simulink model "QuadControlSim"  (R2024b)
settings: Solver=FixedStepAuto  StartTime=0.0  StopTime=15  FixedStep=0.005  RelTol=1e-3
InitFcn:
  | R = 10; % Test Variable
values from neighbouring files (symbols this model uses):
  k = reshape(k,3,6)    [Initialization.m]
  p_Ref = trajMinSnap.p    [Initialization.m]
  psi_Ref = trajMinSnap.psi .* 180/pi    [Initialization.m]
  quad_X500 = quad_X500    [Initialization.m]
  t_Vec = trajMinSnap.t    [Initialization.m]
undefined symbols (not defined in the file or in its folder): kTemp
libraries: slpidlib x6, aerolibconvert2 x3, shared6dof x1, aerolibanimutils x1
settings Model: Creator=tdawg  LastModifiedBy=tdawg
settings SolverCC: ZeroCrossAlgorithm=Adaptive
settings DataIOCC: ReturnWorkspaceOutputs=off
settings DebuggingCC: IgnoredZcDiagnostic=none

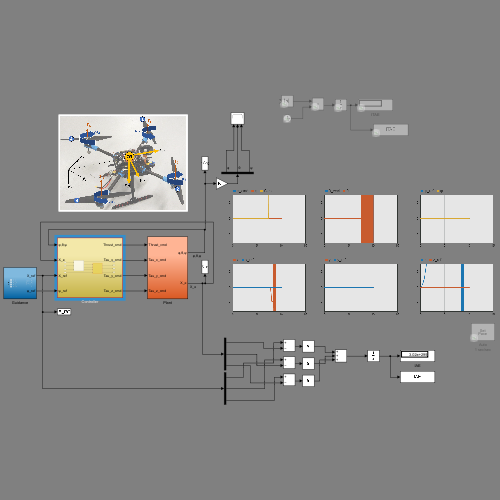
[thumbnail: Simulink's stored preview of the top-level diagram]
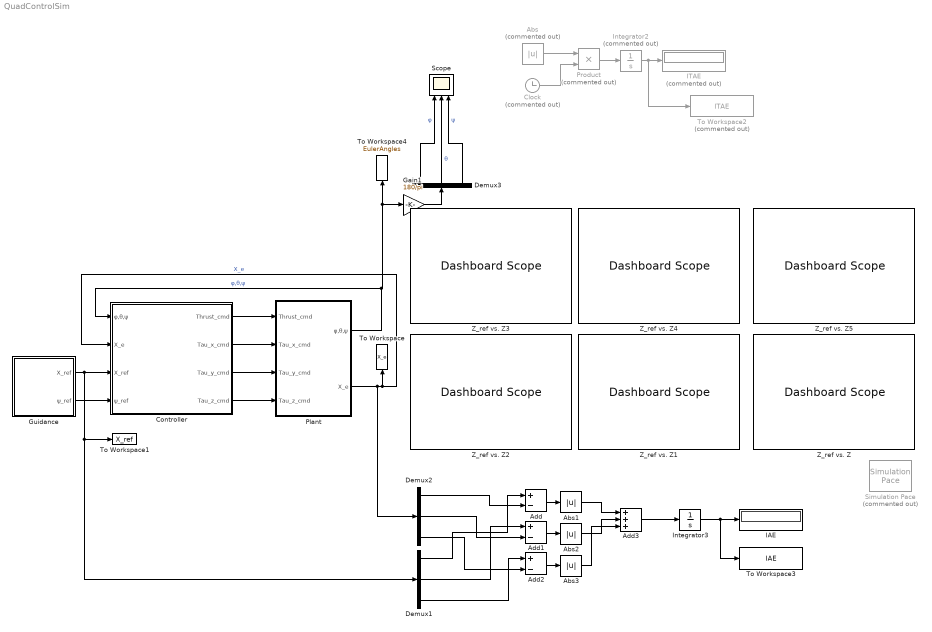
== system QuadControlSim ==
  Abs : Abs  Commented=on  SaturateOnIntegerOverflow=off
  Abs1 : Abs  SaturateOnIntegerOverflow=off
  Abs2 : Abs  SaturateOnIntegerOverflow=off
  Abs3 : Abs  SaturateOnIntegerOverflow=off
  Add : Sum  Inputs=+-
  Add1 : Sum  Inputs=+-
  Add2 : Sum  Inputs=+-
  Add3 : Sum  Inputs=+++
  Clock : Clock  Commented=on
  Controller : Subsystem
  Demux1 : Demux  Outputs=3
  Demux2 : Demux  Outputs=3
  Demux3 : Demux  Outputs=3
  Gain1 : Gain  Gain=180/pi
  Guidance : Subsystem
  IAE : Display
  ITAE : Display  Commented=on
  Integrator2 : Integrator  Commented=on
  Integrator3 : Integrator
  Plant : Subsystem
  Product : Product  Commented=on
  Scope : Scope  NumInputPorts=3
  Simulation Pace : aerolibanimutils/Simulation Pace  Commented=on  SimulationPace=1  SleepMode=Auto  OutputPaceError=off  SampleTime=1/200
  To Workspace : ToWorkspace  VariableName=X_e  SampleTime=-1
  To Workspace1 : ToWorkspace  VariableName=X_ref  SampleTime=-1
  To Workspace2 : ToWorkspace  Commented=on  VariableName=ITAE  SampleTime=-1
  To Workspace3 : ToWorkspace  VariableName=IAE  SampleTime=-1
  To Workspace4 : ToWorkspace  VariableName=EulerAngles  SampleTime=-1
  Z_ref vs. Z{,1..5} (6 alike) : DashboardScope
  wires:
  Guidance/2(ψ_ref) -> Controller/4(ψ_ref)
  Controller/1(Thrust_cmd) -> Plant/1(Thrust_cmd)
  Controller/2(Tau_x_cmd) -> Plant/2(Tau_x_cmd)
  Controller/3(Tau_y_cmd) -> Plant/3(Tau_y_cmd)
  Controller/4(Tau_z_cmd) -> Plant/4(Tau_z_cmd)
  Plant/1(φ,θ,ψ) -> Controller/1(φ,θ,ψ), To Workspace4/1, Gain1/1  "φ,θ,ψ"
  Plant/2(X_e) -> Demux2/1, Controller/2(X_e), To Workspace/1  "X_e"
  Integrator2/1 -> To Workspace2/1, ITAE/1
  Product/1 -> Integrator2/1
  Abs/1 -> Product/1
  Clock/1 -> Product/2
  Demux3/3 -> Scope/3  "ψ"
  Demux3/2 -> Scope/2  "θ"
  Demux3/1 -> Scope/1  "φ"
  Gain1/1 -> Demux3/1
  Add3/1 -> Integrator3/1
  Integrator3/1 -> To Workspace3/1, IAE/1
  Demux1/3 -> Add2/1
  Demux1/2 -> Add1/1
  Demux1/1 -> Add/1
  Demux2/3 -> Add2/2
  Demux2/2 -> Add1/2
  Demux2/1 -> Add/2
  Guidance/1(X_ref) -> Demux1/1, To Workspace1/1, Controller/3(X_ref)
  Add/1 -> Abs1/1
  Add1/1 -> Abs2/1
  Add2/1 -> Abs3/1
  Abs1/1 -> Add3/1
  Abs2/1 -> Add3/2
  Abs3/1 -> Add3/3

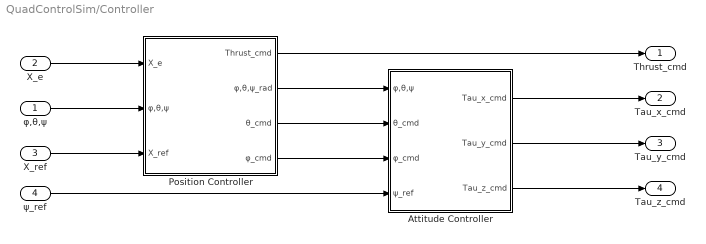
== system QuadControlSim/Controller ==
  φ,θ,ψ : Inport
  X_e : Inport  Port=2
  X_ref : Inport  Port=3
  ψ_ref : Inport  Port=4
  Attitude Controller : Subsystem
  Position Controller : Subsystem
  Thrust_cmd : Outport
  Tau_x_cmd : Outport  Port=2
  Tau_y_cmd : Outport  Port=3
  Tau_z_cmd : Outport  Port=4
  wires:
  Position Controller/4(φ_cmd) -> Attitude Controller/3(φ_cmd)
  Position Controller/2(φ,θ,ψ_rad) -> Attitude Controller/1(φ,θ,ψ)
  Position Controller/3(θ_cmd) -> Attitude Controller/2(θ_cmd)
  Position Controller/1(Thrust_cmd) -> Thrust_cmd/1
  Attitude Controller/1(Tau_x_cmd) -> Tau_x_cmd/1
  Attitude Controller/2(Tau_y_cmd) -> Tau_y_cmd/1
  Attitude Controller/3(Tau_z_cmd) -> Tau_z_cmd/1
  X_e/1 -> Position Controller/1(X_e)
  φ,θ,ψ/1 -> Position Controller/2(φ,θ,ψ)
  X_ref/1 -> Position Controller/3(X_ref)
  ψ_ref/1 -> Attitude Controller/4(ψ_ref)

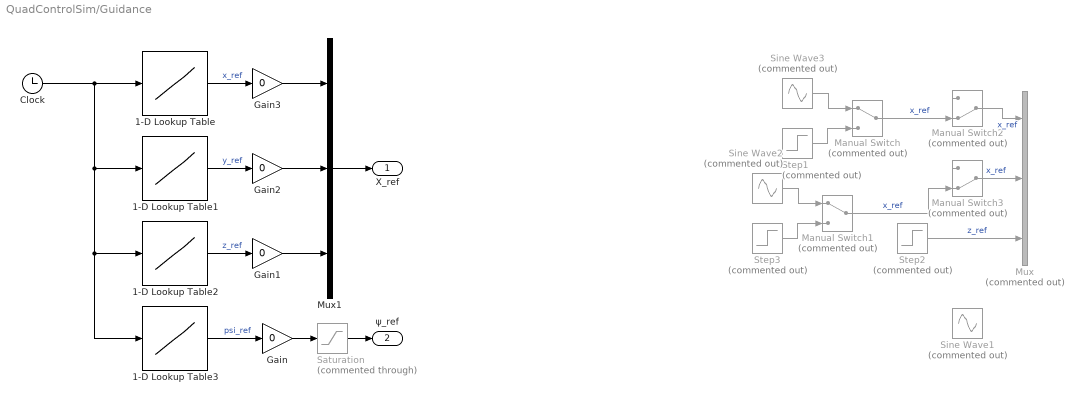
== system QuadControlSim/Guidance ==
  1-D Lookup Table : Lookup_n-D  NumberOfTableDimensions=1  BreakpointsForDimension1=t_Vec  Table=p_Ref(1,:)  InternalRulePriority=Speed  RndMeth=Simplest
  1-D Lookup Table1 : Lookup_n-D  NumberOfTableDimensions=1  BreakpointsForDimension1=t_Vec  Table=p_Ref(2,:)  InternalRulePriority=Speed  RndMeth=Simplest
  1-D Lookup Table2 : Lookup_n-D  NumberOfTableDimensions=1  BreakpointsForDimension1=t_Vec  Table=p_Ref(3,:)  InternalRulePriority=Speed  RndMeth=Simplest
  1-D Lookup Table3 : Lookup_n-D  NumberOfTableDimensions=1  BreakpointsForDimension1=t_Vec  Table=psi_Ref  InternalRulePriority=Speed  RndMeth=Simplest
  Clock : Clock
  Gain{,1..3} (4 alike) : Gain  Gain=0
  Manual Switch : ManualSwitch  Commented=on
  Manual Switch1 : ManualSwitch  Commented=on
  Manual Switch2 : ManualSwitch  Commented=on  CurrentSetting=0
  Manual Switch3 : ManualSwitch  Commented=on  CurrentSetting=0
  Mux : Mux  Commented=on  Inputs=3
  Mux1 : Mux  Inputs=3
  Saturation : Saturate  Commented=through  UpperLimit=175  LowerLimit=-175
  Sine Wave1 : Sin  Commented=on  Amplitude=0  SampleTime=0
  Sine Wave2 : Sin  Commented=on  Frequency=0.5  Phase=pi/2  SampleTime=0
  Sine Wave3 : Sin  Commented=on  Frequency=0.5  SampleTime=0
  Step1 : Step  Commented=on  Time=5  SampleTime=0
  Step2 : Step  Commented=on  After=-2  SampleTime=0
  Step3 : Step  Commented=on  Time=10  SampleTime=0
  X_ref : Outport
  ψ_ref : Outport  Port=2
  wires:
  Step2/1 -> Mux/3  "z_ref"
  Sine Wave3/1 -> Manual Switch/1
  Step1/1 -> Manual Switch/2
  Manual Switch/1 -> Manual Switch2/2  "x_ref"
  Step3/1 -> Manual Switch1/2
  Sine Wave2/1 -> Manual Switch1/1
  Manual Switch1/1 -> Manual Switch3/2  "x_ref"
  Manual Switch2/1 -> Mux/1  "x_ref"
  Manual Switch3/1 -> Mux/2  "x_ref"
  Clock/1 -> 1-D Lookup Table3/1, 1-D Lookup Table2/1, 1-D Lookup Table1/1, 1-D Lookup Table/1
  1-D Lookup Table/1 -> Gain3/1  "x_ref"
  1-D Lookup Table1/1 -> Gain2/1  "y_ref"
  1-D Lookup Table2/1 -> Gain1/1  "z_ref"
  1-D Lookup Table3/1 -> Gain/1  "psi_ref"
  Mux1/1 -> X_ref/1
  Saturation/1 -> ψ_ref/1
  Gain/1 -> Saturation/1
  Gain2/1 -> Mux1/2
  Gain3/1 -> Mux1/1
  Gain1/1 -> Mux1/3

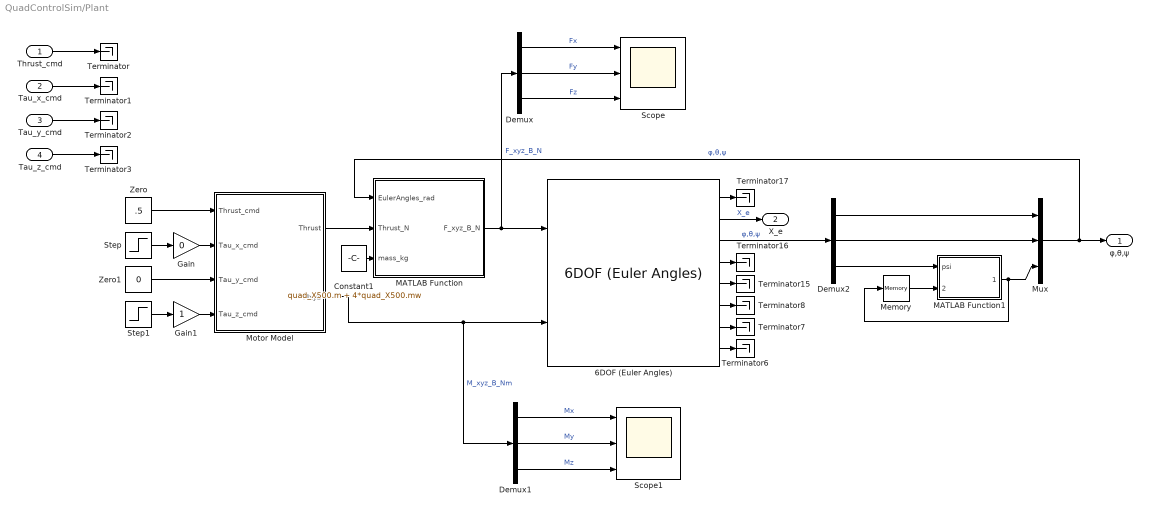
== system QuadControlSim/Plant ==
  Thrust_cmd : Inport
  Tau_x_cmd : Inport  Port=2
  Tau_y_cmd : Inport  Port=3
  Tau_z_cmd : Inport  Port=4
  6DOF (Euler Angles) : shared6dof/6DOF (Euler Angles)  units=Metric (MKS)  mtype=Fixed  rep=Euler Angles  xme_0=[0 0 0]  Vm_0=[0 0 0]  eul_0=[0 0 0]  pm_0=[0 0 0]  mass_0=quad_X500.m + 4*quad_X500.mw  mass_e=0.5  mass_f=2.0  inertia=quad_X500.I  inertia_e=eye(3)  inertia_f=2*eye(3)  k_quat=1  vre_flag=on  abi_flag=off  aMode=0  xme_statename=''  Vm_statename=''  eul_statename=''  quat_statename=''  pm_statename=''  mass_statename=''
  Constant1 : Constant  Value=quad_X500.m + 4*quad_X500.mw
  Demux : Demux  Outputs=3
  Demux1 : Demux  Outputs=3
  Demux2 : Demux  Outputs=3
  Gain : Gain  Gain=0
  Gain1 : Gain
  MATLAB Function : MATLAB Function  TreatAsAtomicUnit=on
  MATLAB Function1 : MATLAB Function  TreatAsAtomicUnit=on
  Memory : Memory
  Motor Model : Subsystem
  Mux : Mux  Inputs=3'
  Scope : Scope  NumInputPorts=3
  Scope1 : Scope  NumInputPorts=3
  Step : Step  Time=7.5  After=0.05  SampleTime=0
  Step1 : Step  Time=7.5  After=0.05  SampleTime=0
  Terminator{,1..3,6..8,15..17} (10 alike) : Terminator
  Zero : Constant  Value=.5  OutDataTypeStr=Inherit: Inherit via back propagation
  Zero1 : Constant  Value=0  OutDataTypeStr=Inherit: Inherit via back propagation
  φ,θ,ψ : Outport
  X_e : Outport  Port=2
  wires:
  6DOF (Euler Angles)/4 -> Terminator16/1
  Constant1/1 -> MATLAB Function/3(mass_kg)
  6DOF (Euler Angles)/6 -> Terminator8/1
  6DOF (Euler Angles)/8 -> Terminator6/1
  MATLAB Function/1(F_xyz_B_N) -> Demux/1, 6DOF (Euler Angles)/1  "F_xyz_B_N"
  6DOF (Euler Angles)/7 -> Terminator7/1
  6DOF (Euler Angles)/5 -> Terminator15/1
  6DOF (Euler Angles)/1 -> Terminator17/1
  6DOF (Euler Angles)/2 -> X_e/1  "X_e"
  Motor Model/1(Thrust) -> MATLAB Function/2(Thrust_N)
  Motor Model/2(Mxyz) -> Demux1/1, 6DOF (Euler Angles)/2  "M_xyz_B_Nm"
  Demux/1 -> Scope/1  "Fx"
  Demux/2 -> Scope/2  "Fy"
  Demux/3 -> Scope/3  "Fz"
  Demux1/1 -> Scope1/1  "Mx"
  Demux1/2 -> Scope1/2  "My"
  Demux1/3 -> Scope1/3  "Mz"
  Demux2/3 -> MATLAB Function1/1(psi)
  MATLAB Function1/1(psi_corrected) -> Mux/3, Memory/1
  Memory/1 -> MATLAB Function1/2(psi_prev)
  6DOF (Euler Angles)/3 -> Demux2/1  "φ,θ,ψ"
  Demux2/2 -> Mux/2
  Demux2/1 -> Mux/1
  Mux/1 -> MATLAB Function/1(EulerAngles_rad), φ,θ,ψ/1  "φ,θ,ψ"
  Thrust_cmd/1 -> Terminator/1
  Tau_x_cmd/1 -> Terminator1/1
  Tau_y_cmd/1 -> Terminator2/1
  Tau_z_cmd/1 -> Terminator3/1
  Zero/1 -> Motor Model/1(Thrust_cmd)
  Zero1/1 -> Motor Model/3(Tau_y_cmd)
  Step/1 -> Gain/1
  Gain/1 -> Motor Model/2(Tau_x_cmd)
  Step1/1 -> Gain1/1
  Gain1/1 -> Motor Model/4(Tau_z_cmd)

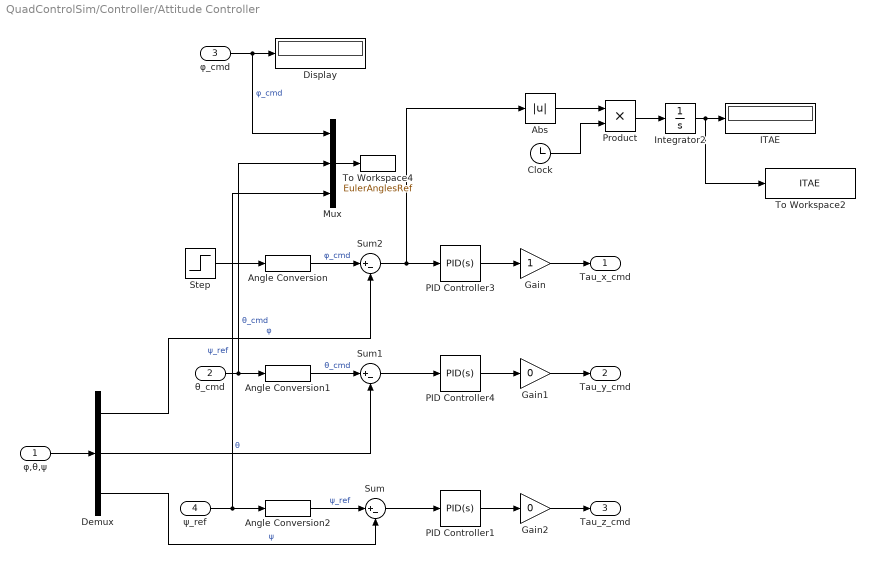
== system QuadControlSim/Controller/Attitude Controller ==
  φ,θ,ψ : Inport
  θ_cmd : Inport  Port=2
  φ_cmd : Inport  Port=3
  ψ_ref : Inport  Port=4
  Abs : Abs  SaturateOnIntegerOverflow=off
  Angle Conversion : aerolibconvert2/Angle Conversion  IU=deg  OU=rad
  Angle Conversion1 : aerolibconvert2/Angle Conversion  IU=deg  OU=rad
  Angle Conversion2 : aerolibconvert2/Angle Conversion  IU=deg  OU=rad
  Clock : Clock
  Demux : Demux  Outputs=3
  Display : Display
  Gain : Gain
  Gain1 : Gain  Gain=0
  Gain2 : Gain  Gain=0
  ITAE : Display
  Integrator2 : Integrator
  Mux : Mux  Inputs=3
  PID Controller1 : slpidlib/PID Controller  Controller=PID  Form=Parallel  TimeDomain=Continuous-time  UseExternalTs=off  SampleTime=-1  IntegratorMethod=Forward Euler  FilterMethod=Forward Euler  ControllerParametersSource=internal  P=k(1,3)  I=k(2,3)  UseKiTs=off  D=k(3,3)  UseExternalDerivativeSource=off  N=100  UseFilter=on  TunerSelectOption=Transfer Function Based (PID Tuner App)  InitialConditionSource=internal  InitialConditionForIntegrator=0  InitialConditionForFilter=0  DifferentiatorICPrevScaledInput=0  ExternalReset=none  TrackingMode=off  Kt=1  LimitOutput=on  SatLimitsSource=internal  UpperSaturationLimit=0.07  LowerSaturationLimit=-0.07  LinearizeAsGain=off  AntiWindupMode=clamping  Kb=0.25  LimitIntegrator=off  UpperIntegratorSaturationLimit=inf  LowerIntegratorSaturationLimit=-inf  POutMin=[]  POutMax=[]  IOutMin=[]  IOutMax=[]  DOutMin=[]  DOutMax=[]  NOutMin=[]  NOutMax=[]  SumOutMin=[]  SumOutMax=[]  SaturationOutMin=[]  SaturationOutMax=[]  PParamMin=[]  PParamMax=[]  IParamMin=[]  IParamMax=[]  DParamMin=[]  DParamMax=[]  NParamMin=[]  NParamMax=[]  KbParamMin=[]  KbParamMax=[]  KtParamMin=[]  KtParamMax=[]  KbOutMin=[]  KbOutMax=[]  KtOutMin=[]  KtOutMax=[]  IntegratorOutMin=[]  IntegratorOutMax=[]  FilterOutMin=[]  FilterOutMax=[]  SumI1OutMin=[]  SumI1OutMax=[]  SumI2OutMin=[]  SumI2OutMax=[]  SumI3OutMin=[]  SumI3OutMax=[]  SumI4OutMin=[]  SumI4OutMax=[]  SumDOutMin=[]  SumDOutMax=[]  DifferentiatorOutMin=[]  DifferentiatorOutMax=[]  FilterDiffOutCoefMin=[]  FilterDiffOutCoefMax=[]  ReciprocalOutMin=[]  ReciprocalOutMax=[]  SumDenOutMin=[]  SumDenOutMax=[]  SumNumOutMin=[]  SumNumOutMax=[]  DivideOutMin=[]  DivideOutMax=[]  UdiffTsProdOutMin=[]  UdiffTsProdOutMax=[]  NTsProdOutMin=[]  NTsProdOutMax=[]  UintegralTsProdOutMin=[]  UintegralTsProdOutMax=[]  UngainTsProdOutMin=[]  UngainTsProdOutMax=[]  ClampingZeroOutDataTypeStr=Inherit: Inherit via back propagation  ClampingZeroOutMin=[]  ClampingZeroOutMax=[]  FilterDenConstantOutDataTypeStr=Inherit: Inherit via back propagation  FilterDenConstantOutMin=[]  FilterDenConstantOutMax=[]  PCopyOutDataTypeStr=Inherit: Inherit via back propagation  PCopyOutMin=[]  PCopyOutMax=[]  NCopyOutDataTypeStr=Inherit: Inherit via back propagation  NCopyOutMin=[]  NCopyOutMax=[]  IntegratorContinuousStateAttributes=''  IntegratorStateMustResolveToSignalObject=off  IntegratorRTWStateStorageClass=Auto  FilterContinuousStateAttributes=''  FilterStateMustResolveToSignalObject=off  FilterRTWStateStorageClass=Auto  ParallelPVariant=InternalParameters  IdealPVariant=Disabled  IVariant=InternalParameters  DVariant=InternalParameters  IntegratorVariant=Continuous  SatVariant=Enabled  AWVariant=ContClampingParallel  PCopyVariant=Disabled  TRVariant=Disabled  FdbkBlocksVariant=Forward  IdealPFdbkVariant=Disabled  SatFdbkVariant=Disabled  DerivativeFilterVariant=ContFilter  NVariant=InternalParameters  NCopyVariant=Disabled  FilterICVariant=InternalICsFilter  IntegratorICVariant=InternalICs  ExternalResetVariant=Disabled  TRSumVariant=Passthrough  SumFdbkVariant=Disabled  SumVariant=Sum_PID  TsampFilterVariant=InternalTs  TsampNgainVariant=Passthrough  TsampIntegralVariant=Disabled_SignalSpec  ExternalSaturationOutDataTypeStr=Inherit: Same as second input  DerivativeSourceVariant=ErrorSignal  PreIntVariant=InternalPreInt
  PID Controller3 : slpidlib/PID Controller  Controller=PID  Form=Parallel  TimeDomain=Continuous-time  UseExternalTs=off  SampleTime=-1  IntegratorMethod=Forward Euler  FilterMethod=Forward Euler  ControllerParametersSource=internal  P=kTemp(1)  I=kTemp(2)  UseKiTs=off  D=kTemp(3)  UseExternalDerivativeSource=off  N=100  UseFilter=on  TunerSelectOption=Transfer Function Based (PID Tuner App)  InitialConditionSource=internal  InitialConditionForIntegrator=0  InitialConditionForFilter=0  DifferentiatorICPrevScaledInput=0  ExternalReset=none  TrackingMode=off  Kt=1  LimitOutput=on  SatLimitsSource=internal  UpperSaturationLimit=0.05  LowerSaturationLimit=-0.05  LinearizeAsGain=off  AntiWindupMode=clamping  Kb=0.25  LimitIntegrator=off  UpperIntegratorSaturationLimit=inf  LowerIntegratorSaturationLimit=-inf  POutMin=[]  POutMax=[]  IOutMin=[]  IOutMax=[]  DOutMin=[]  DOutMax=[]  NOutMin=[]  NOutMax=[]  SumOutMin=[]  SumOutMax=[]  SaturationOutMin=[]  SaturationOutMax=[]  PParamMin=[]  PParamMax=[]  IParamMin=[]  IParamMax=[]  DParamMin=[]  DParamMax=[]  NParamMin=[]  NParamMax=[]  KbParamMin=[]  KbParamMax=[]  KtParamMin=[]  KtParamMax=[]  KbOutMin=[]  KbOutMax=[]  KtOutMin=[]  KtOutMax=[]  IntegratorOutMin=[]  IntegratorOutMax=[]  FilterOutMin=[]  FilterOutMax=[]  SumI1OutMin=[]  SumI1OutMax=[]  SumI2OutMin=[]  SumI2OutMax=[]  SumI3OutMin=[]  SumI3OutMax=[]  SumI4OutMin=[]  SumI4OutMax=[]  SumDOutMin=[]  SumDOutMax=[]  DifferentiatorOutMin=[]  DifferentiatorOutMax=[]  FilterDiffOutCoefMin=[]  FilterDiffOutCoefMax=[]  ReciprocalOutMin=[]  ReciprocalOutMax=[]  SumDenOutMin=[]  SumDenOutMax=[]  SumNumOutMin=[]  SumNumOutMax=[]  DivideOutMin=[]  DivideOutMax=[]  UdiffTsProdOutMin=[]  UdiffTsProdOutMax=[]  NTsProdOutMin=[]  NTsProdOutMax=[]  UintegralTsProdOutMin=[]  UintegralTsProdOutMax=[]  UngainTsProdOutMin=[]  UngainTsProdOutMax=[]  ClampingZeroOutDataTypeStr=Inherit: Inherit via back propagation  ClampingZeroOutMin=[]  ClampingZeroOutMax=[]  FilterDenConstantOutDataTypeStr=Inherit: Inherit via back propagation  FilterDenConstantOutMin=[]  FilterDenConstantOutMax=[]  PCopyOutDataTypeStr=Inherit: Inherit via back propagation  PCopyOutMin=[]  PCopyOutMax=[]  NCopyOutDataTypeStr=Inherit: Inherit via back propagation  NCopyOutMin=[]  NCopyOutMax=[]  IntegratorContinuousStateAttributes=''  IntegratorStateMustResolveToSignalObject=off  IntegratorRTWStateStorageClass=Auto  FilterContinuousStateAttributes=''  FilterStateMustResolveToSignalObject=off  FilterRTWStateStorageClass=Auto  ParallelPVariant=InternalParameters  IdealPVariant=Disabled  IVariant=InternalParameters  DVariant=InternalParameters  IntegratorVariant=Continuous  SatVariant=Enabled  AWVariant=ContClampingParallel  PCopyVariant=Disabled  TRVariant=Disabled  FdbkBlocksVariant=Forward  IdealPFdbkVariant=Disabled  SatFdbkVariant=Disabled  DerivativeFilterVariant=ContFilter  NVariant=InternalParameters  NCopyVariant=Disabled  FilterICVariant=InternalICsFilter  IntegratorICVariant=InternalICs  ExternalResetVariant=Disabled  TRSumVariant=Passthrough  SumFdbkVariant=Disabled  SumVariant=Sum_PID  TsampFilterVariant=InternalTs  TsampNgainVariant=Passthrough  TsampIntegralVariant=Disabled_SignalSpec  ExternalSaturationOutDataTypeStr=Inherit: Same as second input  DerivativeSourceVariant=ErrorSignal  PreIntVariant=InternalPreInt
  PID Controller4 : slpidlib/PID Controller  Controller=PID  Form=Parallel  TimeDomain=Continuous-time  UseExternalTs=off  SampleTime=-1  IntegratorMethod=Forward Euler  FilterMethod=Forward Euler  ControllerParametersSource=internal  P=k(1,2)  I=k(2,2)  UseKiTs=off  D=k(3,2)  UseExternalDerivativeSource=off  N=100  UseFilter=on  TunerSelectOption=Transfer Function Based (PID Tuner App)  InitialConditionSource=internal  InitialConditionForIntegrator=0  InitialConditionForFilter=0  DifferentiatorICPrevScaledInput=0  ExternalReset=none  TrackingMode=off  Kt=1  LimitOutput=on  SatLimitsSource=internal  UpperSaturationLimit=0.05  LowerSaturationLimit=-0.05  LinearizeAsGain=off  AntiWindupMode=clamping  Kb=0.25  LimitIntegrator=off  UpperIntegratorSaturationLimit=inf  LowerIntegratorSaturationLimit=-inf  POutMin=[]  POutMax=[]  IOutMin=[]  IOutMax=[]  DOutMin=[]  DOutMax=[]  NOutMin=[]  NOutMax=[]  SumOutMin=[]  SumOutMax=[]  SaturationOutMin=[]  SaturationOutMax=[]  PParamMin=[]  PParamMax=[]  IParamMin=[]  IParamMax=[]  DParamMin=[]  DParamMax=[]  NParamMin=[]  NParamMax=[]  KbParamMin=[]  KbParamMax=[]  KtParamMin=[]  KtParamMax=[]  KbOutMin=[]  KbOutMax=[]  KtOutMin=[]  KtOutMax=[]  IntegratorOutMin=[]  IntegratorOutMax=[]  FilterOutMin=[]  FilterOutMax=[]  SumI1OutMin=[]  SumI1OutMax=[]  SumI2OutMin=[]  SumI2OutMax=[]  SumI3OutMin=[]  SumI3OutMax=[]  SumI4OutMin=[]  SumI4OutMax=[]  SumDOutMin=[]  SumDOutMax=[]  DifferentiatorOutMin=[]  DifferentiatorOutMax=[]  FilterDiffOutCoefMin=[]  FilterDiffOutCoefMax=[]  ReciprocalOutMin=[]  ReciprocalOutMax=[]  SumDenOutMin=[]  SumDenOutMax=[]  SumNumOutMin=[]  SumNumOutMax=[]  DivideOutMin=[]  DivideOutMax=[]  UdiffTsProdOutMin=[]  UdiffTsProdOutMax=[]  NTsProdOutMin=[]  NTsProdOutMax=[]  UintegralTsProdOutMin=[]  UintegralTsProdOutMax=[]  UngainTsProdOutMin=[]  UngainTsProdOutMax=[]  ClampingZeroOutDataTypeStr=Inherit: Inherit via back propagation  ClampingZeroOutMin=[]  ClampingZeroOutMax=[]  FilterDenConstantOutDataTypeStr=Inherit: Inherit via back propagation  FilterDenConstantOutMin=[]  FilterDenConstantOutMax=[]  PCopyOutDataTypeStr=Inherit: Inherit via back propagation  PCopyOutMin=[]  PCopyOutMax=[]  NCopyOutDataTypeStr=Inherit: Inherit via back propagation  NCopyOutMin=[]  NCopyOutMax=[]  IntegratorContinuousStateAttributes=''  IntegratorStateMustResolveToSignalObject=off  IntegratorRTWStateStorageClass=Auto  FilterContinuousStateAttributes=''  FilterStateMustResolveToSignalObject=off  FilterRTWStateStorageClass=Auto  ParallelPVariant=InternalParameters  IdealPVariant=Disabled  IVariant=InternalParameters  DVariant=InternalParameters  IntegratorVariant=Continuous  SatVariant=Enabled  AWVariant=ContClampingParallel  PCopyVariant=Disabled  TRVariant=Disabled  FdbkBlocksVariant=Forward  IdealPFdbkVariant=Disabled  SatFdbkVariant=Disabled  DerivativeFilterVariant=ContFilter  NVariant=InternalParameters  NCopyVariant=Disabled  FilterICVariant=InternalICsFilter  IntegratorICVariant=InternalICs  ExternalResetVariant=Disabled  TRSumVariant=Passthrough  SumFdbkVariant=Disabled  SumVariant=Sum_PID  TsampFilterVariant=InternalTs  TsampNgainVariant=Passthrough  TsampIntegralVariant=Disabled_SignalSpec  ExternalSaturationOutDataTypeStr=Inherit: Same as second input  DerivativeSourceVariant=ErrorSignal  PreIntVariant=InternalPreInt
  Product : Product
  Step : Step  Time=7.5  After=10  SampleTime=0
  Sum : Sum  Inputs=|+-
  Sum1 : Sum  Inputs=|+-
  Sum2 : Sum  Inputs=|+-
  To Workspace2 : ToWorkspace  VariableName=ITAE  SampleTime=-1
  To Workspace4 : ToWorkspace  VariableName=EulerAnglesRef  SampleTime=-1
  Tau_x_cmd : Outport
  Tau_y_cmd : Outport  Port=2
  Tau_z_cmd : Outport  Port=3
  wires:
  Sum/1 -> PID Controller1/1
  Demux/3 -> Sum/2  "ψ"
  Sum1/1 -> PID Controller4/1
  Sum2/1 -> Abs/1, PID Controller3/1
  Demux/2 -> Sum1/2  "θ"
  Demux/1 -> Sum2/2  "φ"
  φ,θ,ψ/1 -> Demux/1
  PID Controller3/1 -> Gain/1
  PID Controller4/1 -> Gain1/1
  PID Controller1/1 -> Gain2/1
  Angle Conversion/1 -> Sum2/1  "φ_cmd"
  Angle Conversion1/1 -> Sum1/1  "θ_cmd"
  Angle Conversion2/1 -> Sum/1  "ψ_ref"
  Mux/1 -> To Workspace4/1
  θ_cmd/1 -> Angle Conversion1/1, Mux/2  "θ_cmd"
  ψ_ref/1 -> Angle Conversion2/1, Mux/3  "ψ_ref"
  Gain/1 -> Tau_x_cmd/1
  Gain1/1 -> Tau_y_cmd/1
  Gain2/1 -> Tau_z_cmd/1
  Clock/1 -> Product/2
  Product/1 -> Integrator2/1
  Abs/1 -> Product/1
  Integrator2/1 -> To Workspace2/1, ITAE/1
  φ_cmd/1 -> Mux/1, Display/1  "φ_cmd"
  Step/1 -> Angle Conversion/1

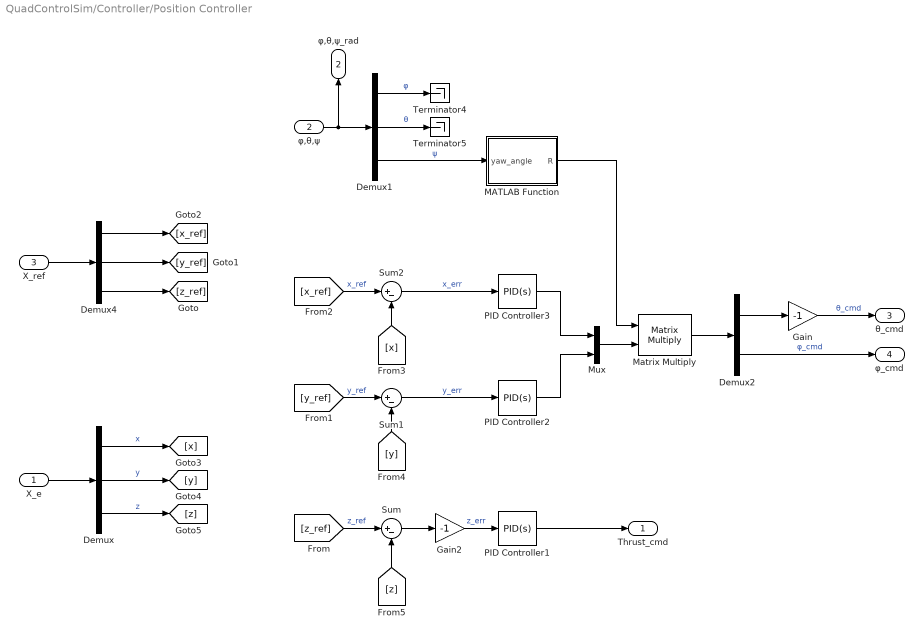
== system QuadControlSim/Controller/Position Controller ==
  X_e : Inport
  φ,θ,ψ : Inport  Port=2
  X_ref : Inport  Port=3
  Demux : Demux  Outputs=3
  Demux1 : Demux  Outputs=3
  Demux2 : Demux  Outputs=2
  Demux4 : Demux  Outputs=3
  Gain : Gain  Gain=-1
  Gain2 : Gain  Gain=-1
  MATLAB Function : MATLAB Function  TreatAsAtomicUnit=on
  Matrix Multiply : Product  Multiplication=Matrix(*)
  Mux : Mux  Inputs=2
  PID Controller1 : slpidlib/PID Controller  Controller=PID  Form=Parallel  TimeDomain=Continuous-time  UseExternalTs=off  SampleTime=-1  IntegratorMethod=Forward Euler  FilterMethod=Forward Euler  ControllerParametersSource=internal  P=k(1,6)  I=k(2,6)  UseKiTs=off  D=k(3,6)  UseExternalDerivativeSource=off  N=100  UseFilter=on  TunerSelectOption=Transfer Function Based (PID Tuner App)  InitialConditionSource=internal  InitialConditionForIntegrator=0  InitialConditionForFilter=0  DifferentiatorICPrevScaledInput=0  ExternalReset=none  TrackingMode=off  Kt=1  LimitOutput=on  SatLimitsSource=internal  UpperSaturationLimit=1  LowerSaturationLimit=0  LinearizeAsGain=off  AntiWindupMode=back-calculation  Kb=0.25  LimitIntegrator=off  UpperIntegratorSaturationLimit=inf  LowerIntegratorSaturationLimit=-inf  POutMin=[]  POutMax=[]  IOutMin=[]  IOutMax=[]  DOutMin=[]  DOutMax=[]  NOutMin=[]  NOutMax=[]  SumOutMin=[]  SumOutMax=[]  SaturationOutMin=[]  SaturationOutMax=[]  PParamMin=[]  PParamMax=[]  IParamMin=[]  IParamMax=[]  DParamMin=[]  DParamMax=[]  NParamMin=[]  NParamMax=[]  KbParamMin=[]  KbParamMax=[]  KtParamMin=[]  KtParamMax=[]  KbOutMin=[]  KbOutMax=[]  KtOutMin=[]  KtOutMax=[]  IntegratorOutMin=[]  IntegratorOutMax=[]  FilterOutMin=[]  FilterOutMax=[]  SumI1OutMin=[]  SumI1OutMax=[]  SumI2OutMin=[]  SumI2OutMax=[]  SumI3OutMin=[]  SumI3OutMax=[]  SumI4OutMin=[]  SumI4OutMax=[]  SumDOutMin=[]  SumDOutMax=[]  DifferentiatorOutMin=[]  DifferentiatorOutMax=[]  FilterDiffOutCoefMin=[]  FilterDiffOutCoefMax=[]  ReciprocalOutMin=[]  ReciprocalOutMax=[]  SumDenOutMin=[]  SumDenOutMax=[]  SumNumOutMin=[]  SumNumOutMax=[]  DivideOutMin=[]  DivideOutMax=[]  UdiffTsProdOutMin=[]  UdiffTsProdOutMax=[]  NTsProdOutMin=[]  NTsProdOutMax=[]  UintegralTsProdOutMin=[]  UintegralTsProdOutMax=[]  UngainTsProdOutMin=[]  UngainTsProdOutMax=[]  ClampingZeroOutDataTypeStr=Inherit: Inherit via back propagation  ClampingZeroOutMin=[]  ClampingZeroOutMax=[]  FilterDenConstantOutDataTypeStr=Inherit: Inherit via back propagation  FilterDenConstantOutMin=[]  FilterDenConstantOutMax=[]  PCopyOutDataTypeStr=Inherit: Inherit via back propagation  PCopyOutMin=[]  PCopyOutMax=[]  NCopyOutDataTypeStr=Inherit: Inherit via back propagation  NCopyOutMin=[]  NCopyOutMax=[]  IntegratorContinuousStateAttributes=''  IntegratorStateMustResolveToSignalObject=off  IntegratorRTWStateStorageClass=Auto  FilterContinuousStateAttributes=''  FilterStateMustResolveToSignalObject=off  FilterRTWStateStorageClass=Auto  ParallelPVariant=InternalParameters  IdealPVariant=Disabled  IVariant=InternalParameters  DVariant=InternalParameters  IntegratorVariant=Continuous  SatVariant=Enabled  AWVariant=BackCalculation  PCopyVariant=Disabled  TRVariant=Disabled  FdbkBlocksVariant=Forward  IdealPFdbkVariant=Disabled  SatFdbkVariant=Disabled  DerivativeFilterVariant=ContFilter  NVariant=InternalParameters  NCopyVariant=Disabled  FilterICVariant=InternalICsFilter  IntegratorICVariant=InternalICs  ExternalResetVariant=Disabled  TRSumVariant=Passthrough  SumFdbkVariant=Disabled  SumVariant=Sum_PID  TsampFilterVariant=InternalTs  TsampNgainVariant=Passthrough  TsampIntegralVariant=Disabled_SignalSpec  ExternalSaturationOutDataTypeStr=Inherit: Same as second input  DerivativeSourceVariant=ErrorSignal  PreIntVariant=InternalPreInt
  PID Controller2 : slpidlib/PID Controller  Controller=PID  Form=Parallel  TimeDomain=Continuous-time  UseExternalTs=off  SampleTime=-1  IntegratorMethod=Forward Euler  FilterMethod=Forward Euler  ControllerParametersSource=internal  P=k(1,5)  I=k(2,5)  UseKiTs=off  D=k(3,5)  UseExternalDerivativeSource=off  N=100  UseFilter=on  TunerSelectOption=Transfer Function Based (PID Tuner App)  InitialConditionSource=internal  InitialConditionForIntegrator=0  InitialConditionForFilter=0  DifferentiatorICPrevScaledInput=0  ExternalReset=none  TrackingMode=off  Kt=1  LimitOutput=on  SatLimitsSource=internal  UpperSaturationLimit=15  LowerSaturationLimit=-15  LinearizeAsGain=off  AntiWindupMode=clamping  Kb=0.25  LimitIntegrator=off  UpperIntegratorSaturationLimit=inf  LowerIntegratorSaturationLimit=-inf  POutMin=[]  POutMax=[]  IOutMin=[]  IOutMax=[]  DOutMin=[]  DOutMax=[]  NOutMin=[]  NOutMax=[]  SumOutMin=[]  SumOutMax=[]  SaturationOutMin=[]  SaturationOutMax=[]  PParamMin=[]  PParamMax=[]  IParamMin=[]  IParamMax=[]  DParamMin=[]  DParamMax=[]  NParamMin=[]  NParamMax=[]  KbParamMin=[]  KbParamMax=[]  KtParamMin=[]  KtParamMax=[]  KbOutMin=[]  KbOutMax=[]  KtOutMin=[]  KtOutMax=[]  IntegratorOutMin=[]  IntegratorOutMax=[]  FilterOutMin=[]  FilterOutMax=[]  SumI1OutMin=[]  SumI1OutMax=[]  SumI2OutMin=[]  SumI2OutMax=[]  SumI3OutMin=[]  SumI3OutMax=[]  SumI4OutMin=[]  SumI4OutMax=[]  SumDOutMin=[]  SumDOutMax=[]  DifferentiatorOutMin=[]  DifferentiatorOutMax=[]  FilterDiffOutCoefMin=[]  FilterDiffOutCoefMax=[]  ReciprocalOutMin=[]  ReciprocalOutMax=[]  SumDenOutMin=[]  SumDenOutMax=[]  SumNumOutMin=[]  SumNumOutMax=[]  DivideOutMin=[]  DivideOutMax=[]  UdiffTsProdOutMin=[]  UdiffTsProdOutMax=[]  NTsProdOutMin=[]  NTsProdOutMax=[]  UintegralTsProdOutMin=[]  UintegralTsProdOutMax=[]  UngainTsProdOutMin=[]  UngainTsProdOutMax=[]  ClampingZeroOutDataTypeStr=Inherit: Inherit via back propagation  ClampingZeroOutMin=[]  ClampingZeroOutMax=[]  FilterDenConstantOutDataTypeStr=Inherit: Inherit via back propagation  FilterDenConstantOutMin=[]  FilterDenConstantOutMax=[]  PCopyOutDataTypeStr=Inherit: Inherit via back propagation  PCopyOutMin=[]  PCopyOutMax=[]  NCopyOutDataTypeStr=Inherit: Inherit via back propagation  NCopyOutMin=[]  NCopyOutMax=[]  IntegratorContinuousStateAttributes=''  IntegratorStateMustResolveToSignalObject=off  IntegratorRTWStateStorageClass=Auto  FilterContinuousStateAttributes=''  FilterStateMustResolveToSignalObject=off  FilterRTWStateStorageClass=Auto  ParallelPVariant=InternalParameters  IdealPVariant=Disabled  IVariant=InternalParameters  DVariant=InternalParameters  IntegratorVariant=Continuous  SatVariant=Enabled  AWVariant=ContClampingParallel  PCopyVariant=Disabled  TRVariant=Disabled  FdbkBlocksVariant=Forward  IdealPFdbkVariant=Disabled  SatFdbkVariant=Disabled  DerivativeFilterVariant=ContFilter  NVariant=InternalParameters  NCopyVariant=Disabled  FilterICVariant=InternalICsFilter  IntegratorICVariant=InternalICs  ExternalResetVariant=Disabled  TRSumVariant=Passthrough  SumFdbkVariant=Disabled  SumVariant=Sum_PID  TsampFilterVariant=InternalTs  TsampNgainVariant=Passthrough  TsampIntegralVariant=Disabled_SignalSpec  ExternalSaturationOutDataTypeStr=Inherit: Same as second input  DerivativeSourceVariant=ErrorSignal  PreIntVariant=InternalPreInt
  PID Controller3 : slpidlib/PID Controller  Controller=PID  Form=Parallel  TimeDomain=Continuous-time  UseExternalTs=off  SampleTime=-1  IntegratorMethod=Forward Euler  FilterMethod=Forward Euler  ControllerParametersSource=internal  P=k(1,4)  I=k(2,4)  UseKiTs=off  D=k(3,4)  UseExternalDerivativeSource=off  N=100  UseFilter=on  TunerSelectOption=Transfer Function Based (PID Tuner App)  InitialConditionSource=internal  InitialConditionForIntegrator=0  InitialConditionForFilter=0  DifferentiatorICPrevScaledInput=0  ExternalReset=none  TrackingMode=off  Kt=1  LimitOutput=on  SatLimitsSource=internal  UpperSaturationLimit=15  LowerSaturationLimit=-15  LinearizeAsGain=off  AntiWindupMode=clamping  Kb=0.25  LimitIntegrator=off  UpperIntegratorSaturationLimit=inf  LowerIntegratorSaturationLimit=-inf  POutMin=[]  POutMax=[]  IOutMin=[]  IOutMax=[]  DOutMin=[]  DOutMax=[]  NOutMin=[]  NOutMax=[]  SumOutMin=[]  SumOutMax=[]  SaturationOutMin=[]  SaturationOutMax=[]  PParamMin=[]  PParamMax=[]  IParamMin=[]  IParamMax=[]  DParamMin=[]  DParamMax=[]  NParamMin=[]  NParamMax=[]  KbParamMin=[]  KbParamMax=[]  KtParamMin=[]  KtParamMax=[]  KbOutMin=[]  KbOutMax=[]  KtOutMin=[]  KtOutMax=[]  IntegratorOutMin=[]  IntegratorOutMax=[]  FilterOutMin=[]  FilterOutMax=[]  SumI1OutMin=[]  SumI1OutMax=[]  SumI2OutMin=[]  SumI2OutMax=[]  SumI3OutMin=[]  SumI3OutMax=[]  SumI4OutMin=[]  SumI4OutMax=[]  SumDOutMin=[]  SumDOutMax=[]  DifferentiatorOutMin=[]  DifferentiatorOutMax=[]  FilterDiffOutCoefMin=[]  FilterDiffOutCoefMax=[]  ReciprocalOutMin=[]  ReciprocalOutMax=[]  SumDenOutMin=[]  SumDenOutMax=[]  SumNumOutMin=[]  SumNumOutMax=[]  DivideOutMin=[]  DivideOutMax=[]  UdiffTsProdOutMin=[]  UdiffTsProdOutMax=[]  NTsProdOutMin=[]  NTsProdOutMax=[]  UintegralTsProdOutMin=[]  UintegralTsProdOutMax=[]  UngainTsProdOutMin=[]  UngainTsProdOutMax=[]  ClampingZeroOutDataTypeStr=Inherit: Inherit via back propagation  ClampingZeroOutMin=[]  ClampingZeroOutMax=[]  FilterDenConstantOutDataTypeStr=Inherit: Inherit via back propagation  FilterDenConstantOutMin=[]  FilterDenConstantOutMax=[]  PCopyOutDataTypeStr=Inherit: Inherit via back propagation  PCopyOutMin=[]  PCopyOutMax=[]  NCopyOutDataTypeStr=Inherit: Inherit via back propagation  NCopyOutMin=[]  NCopyOutMax=[]  IntegratorContinuousStateAttributes=''  IntegratorStateMustResolveToSignalObject=off  IntegratorRTWStateStorageClass=Auto  FilterContinuousStateAttributes=''  FilterStateMustResolveToSignalObject=off  FilterRTWStateStorageClass=Auto  ParallelPVariant=InternalParameters  IdealPVariant=Disabled  IVariant=InternalParameters  DVariant=InternalParameters  IntegratorVariant=Continuous  SatVariant=Enabled  AWVariant=ContClampingParallel  PCopyVariant=Disabled  TRVariant=Disabled  FdbkBlocksVariant=Forward  IdealPFdbkVariant=Disabled  SatFdbkVariant=Disabled  DerivativeFilterVariant=ContFilter  NVariant=InternalParameters  NCopyVariant=Disabled  FilterICVariant=InternalICsFilter  IntegratorICVariant=InternalICs  ExternalResetVariant=Disabled  TRSumVariant=Passthrough  SumFdbkVariant=Disabled  SumVariant=Sum_PID  TsampFilterVariant=InternalTs  TsampNgainVariant=Passthrough  TsampIntegralVariant=Disabled_SignalSpec  ExternalSaturationOutDataTypeStr=Inherit: Same as second input  DerivativeSourceVariant=ErrorSignal  PreIntVariant=InternalPreInt
  Sum : Sum  Inputs=|+-
  Sum1 : Sum  Inputs=|+-
  Sum2 : Sum  Inputs=|+-
  Terminator4 : Terminator
  Terminator5 : Terminator
  Thrust_cmd : Outport
  φ,θ,ψ_rad : Outport  Port=2
  θ_cmd : Outport  Port=3
  φ_cmd : Outport  Port=4
  wires:
  X_ref/1 -> Demux4/1
  Demux4/1 -> [x_ref]
  Demux4/2 -> [y_ref]
  Demux4/3 -> [z_ref]
  X_e/1 -> Demux/1
  Demux/1 -> [x]  "x"
  Demux/2 -> [y]  "y"
  Demux/3 -> [z]  "z"
  φ,θ,ψ/1 -> φ,θ,ψ_rad/1, Demux1/1
  Demux1/1 -> Terminator4/1  "φ"
  Demux1/2 -> Terminator5/1  "θ"
  Demux1/3 -> MATLAB Function/1(yaw_angle)  "ψ"
  Sum1/1 -> PID Controller2/1  "y_err"
  Sum2/1 -> PID Controller3/1  "x_err"
  Gain2/1 -> PID Controller1/1  "z_err"
  PID Controller3/1 -> Mux/1
  PID Controller2/1 -> Mux/2
  Mux/1 -> Matrix Multiply/2
  MATLAB Function/1(R) -> Matrix Multiply/1
  Matrix Multiply/1 -> Demux2/1
  Demux2/1 -> Gain/1
  Gain/1 -> θ_cmd/1  "θ_cmd"
  Demux2/2 -> φ_cmd/1  "φ_cmd"
  [x_ref] -> Sum2/1  "x_ref"
  Sum/1 -> Gain2/1
  [y_ref] -> Sum1/1  "y_ref"
  [z_ref] -> Sum/1  "z_ref"
  [x] -> Sum2/2
  [y] -> Sum1/2
  [z] -> Sum/2
  PID Controller1/1 -> Thrust_cmd/1

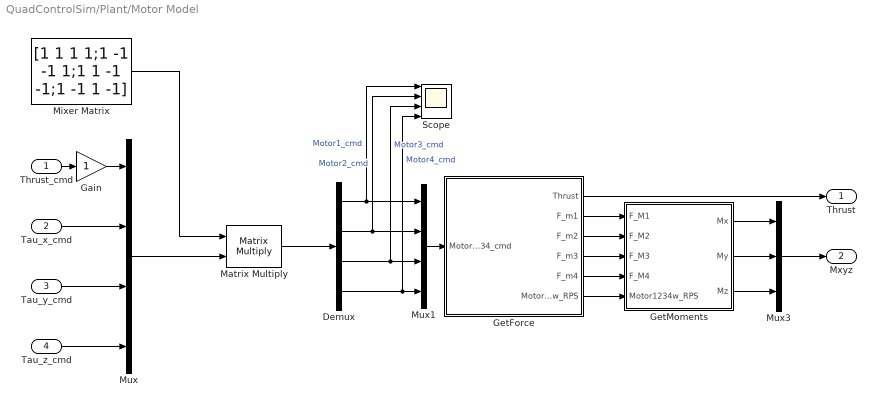
== system QuadControlSim/Plant/Motor Model ==
  Thrust_cmd : Inport
  Tau_x_cmd : Inport  Port=2
  Tau_y_cmd : Inport  Port=3
  Tau_z_cmd : Inport  Port=4
  Demux : Demux
  Gain : Gain
  GetForce : Subsystem
  GetMoments : Subsystem
  Matrix Multiply : Product  Multiplication=Matrix(*)
  Mixer Matrix : Constant  Value=[1 1 1 1;1 -1 -1 1;1 1 -1 -1;1 -1 1 -1]
  Mux : Mux
  Mux1 : Mux
  Mux3 : Mux  Inputs=3
  Scope : Scope  NumInputPorts=4
  Thrust : Outport
  Mxyz : Outport  Port=2
  wires:
  GetForce/1(Thrust) -> Thrust/1
  Mux3/1 -> Mxyz/1
  GetMoments/3(Mz) -> Mux3/3
  GetMoments/1(Mx) -> Mux3/1
  GetMoments/2(My) -> Mux3/2
  GetForce/5(F_m4) -> GetMoments/4(F_M4)
  GetForce/4(F_m3) -> GetMoments/3(F_M3)
  GetForce/3(F_m2) -> GetMoments/2(F_M2)
  GetForce/2(F_m1) -> GetMoments/1(F_M1)
  Mux1/1 -> GetForce/1(Motor1234_cmd)
  Demux/4 -> Scope/4, Mux1/4  "Motor4_cmd"
  Demux/3 -> Scope/3, Mux1/3  "Motor3_cmd"
  Demux/2 -> Scope/2, Mux1/2  "Motor2_cmd"
  Demux/1 -> Scope/1, Mux1/1  "Motor1_cmd"
  Matrix Multiply/1 -> Demux/1
  Mixer Matrix/1 -> Matrix Multiply/1
  Mux/1 -> Matrix Multiply/2
  Thrust_cmd/1 -> Gain/1
  GetForce/6(Motor1234w_RPS) -> GetMoments/5(Motor1234w_RPS)
  Gain/1 -> Mux/1
  Tau_z_cmd/1 -> Mux/4
  Tau_x_cmd/1 -> Mux/2
  Tau_y_cmd/1 -> Mux/3

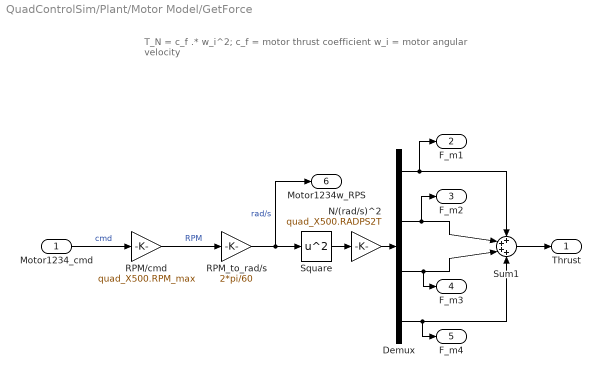
== system QuadControlSim/Plant/Motor Model/GetForce ==
  note: T_N = c_f .* w_i^2;
      | c_f = motor thrust coefficient
      | w_i = motor angular velocity
  Motor1234_cmd : Inport
  Demux : Demux
  N/(rad/s)^2 : Gain  Gain=quad_X500.RADPS2T
  RPM/cmd : Gain  Gain=quad_X500.RPM_max
  RPM_to_rad/s : Gain  Gain=2*pi/60
  Square : Math  Operator=square
  Sum1 : Sum  Inputs=++++
  Thrust : Outport
  F_m1 : Outport  Port=2
  F_m2 : Outport  Port=3
  F_m3 : Outport  Port=4
  F_m4 : Outport  Port=5
  Motor1234w_RPS : Outport  Port=6
  wires:
  Motor1234_cmd/1 -> RPM/cmd/1  "cmd"
  RPM/cmd/1 -> RPM_to_rad/s/1  "RPM"
  RPM_to_rad/s/1 -> Motor1234w_RPS/1, Square/1  "rad/s"
  N/(rad/s)^2/1 -> Demux/1
  Demux/1 -> F_m1/1, Sum1/1
  Demux/2 -> F_m2/1, Sum1/2
  Demux/3 -> F_m3/1, Sum1/3
  Demux/4 -> F_m4/1, Sum1/4
  Sum1/1 -> Thrust/1
  Square/1 -> N/(rad/s)^2/1

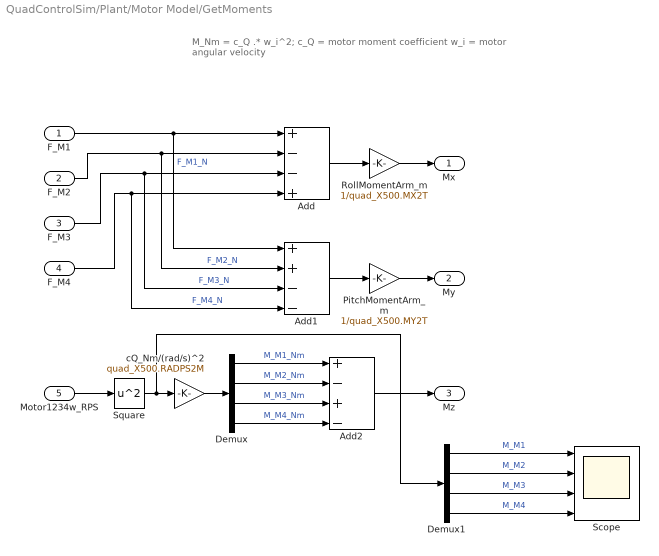
== system QuadControlSim/Plant/Motor Model/GetMoments ==
  note: M_Nm = c_Q .* w_i^2;
      | c_Q = motor moment coefficient
      | w_i = motor angular velocity
  F_M1 : Inport
  F_M2 : Inport  Port=2
  F_M3 : Inport  Port=3
  F_M4 : Inport  Port=4
  Motor1234w_RPS : Inport  Port=5
  Add : Sum  Inputs=+--+
  Add1 : Sum  Inputs=++--
  Add2 : Sum  Inputs=+-+-
  Demux : Demux
  Demux1 : Demux
  PitchMomentArm_m : Gain  Gain=1/quad_X500.MY2T
  RollMomentArm_m : Gain  Gain=1/quad_X500.MX2T
  Scope : Scope  NumInputPorts=4
  Square : Math  Operator=square
  cQ_Nm/(rad/s)^2 : Gain  Gain=quad_X500.RADPS2M
  Mx : Outport
  My : Outport  Port=2
  Mz : Outport  Port=3
  wires:
  F_M1/1 -> Add1/1, Add/1  "F_M1_N"
  F_M2/1 -> Add1/2, Add/2  "F_M2_N"
  F_M3/1 -> Add1/3, Add/3  "F_M3_N"
  Add/1 -> RollMomentArm_m/1
  Add1/1 -> PitchMomentArm_m/1
  F_M4/1 -> Add1/4, Add/4  "F_M4_N"
  RollMomentArm_m/1 -> Mx/1
  PitchMomentArm_m/1 -> My/1
  Add2/1 -> Mz/1
  Motor1234w_RPS/1 -> Square/1
  cQ_Nm/(rad/s)^2/1 -> Demux/1
  Demux/1 -> Add2/1  "M_M1_Nm"
  Demux/2 -> Add2/2  "M_M2_Nm"
  Demux/3 -> Add2/3  "M_M3_Nm"
  Demux/4 -> Add2/4  "M_M4_Nm"
  Square/1 -> Demux1/1, cQ_Nm/(rad/s)^2/1
  Demux1/1 -> Scope/1  "M_M1"
  Demux1/2 -> Scope/2  "M_M2"
  Demux1/3 -> Scope/3  "M_M3"
  Demux1/4 -> Scope/4  "M_M4"

== matlab function QuadControlSim/Plant/MATLAB Function ==
  data: EulerAngles_rad input; F_xyz_B_N output; Thrust_N input; mass_kg input
function F_xyz_B_N = fcn(EulerAngles_rad,Thrust_N,mass_kg) % codegen
phi = EulerAngles_rad(1);
theta = EulerAngles_rad(2);
psi = EulerAngles_rad(3);

Rz = [cos(psi) sin(psi) 0; -sin(psi) cos(psi) 0; 0 0 1];
Ry = [cos(theta) 0 -sin(theta); 0 1 0; sin(theta) 0 cos(theta)];
Rx = [1 0 0; 0 cos(phi) sin(phi); 0 -sin(phi) cos(phi)];

R_ZYX = Rx*Ry*Rz;

F_xyz_B_N = R_ZYX' * [0;0;9.81] .* mass_kg + [0;0;-Thrust_N];
end

== matlab function QuadControlSim/Controller/Position Controller/MATLAB Function ==
  data: yaw_angle input; R output
function R = YawCorrection(yaw_angle) % codegen

R = [cos(yaw_angle) sin(yaw_angle);
     -sin(yaw_angle) cos(yaw_angle)];

== matlab function QuadControlSim/Plant/MATLAB Function1 ==
  data: psi input; psi_corrected output; psi_prev input
function psi_corrected = fcn(psi, psi_prev)
del_psi = psi-psi_prev;
if abs(del_psi)>=pi && del_psi<=pi
    psi_corrected = psi+2*pi;
elseif abs(del_psi)>=pi && del_psi>=pi
    psi_corrected = psi-2*pi;
else
    psi_corrected = psi;
end
